simulink model "RealModelwithFlexibleLoad"  (R2019a)
settings: Solver=ode4  StartTime=0.0  StopTime=50.0  FixedStep=5e-5  MaxStep=1e-4  RelTol=1e-5
InitFcn:
  | Rs = 0.011
  | Ld = 0.018
  | Lq = 0.018
  | Fi = 0.055
  | p = 4
  | J = 0.002
  | b = 0.18
  | JL = 0.10
  | Bs = 0.00
  | Ks = 50
settings Model: Creator=LiLid  LastModifiedBy=LiLid

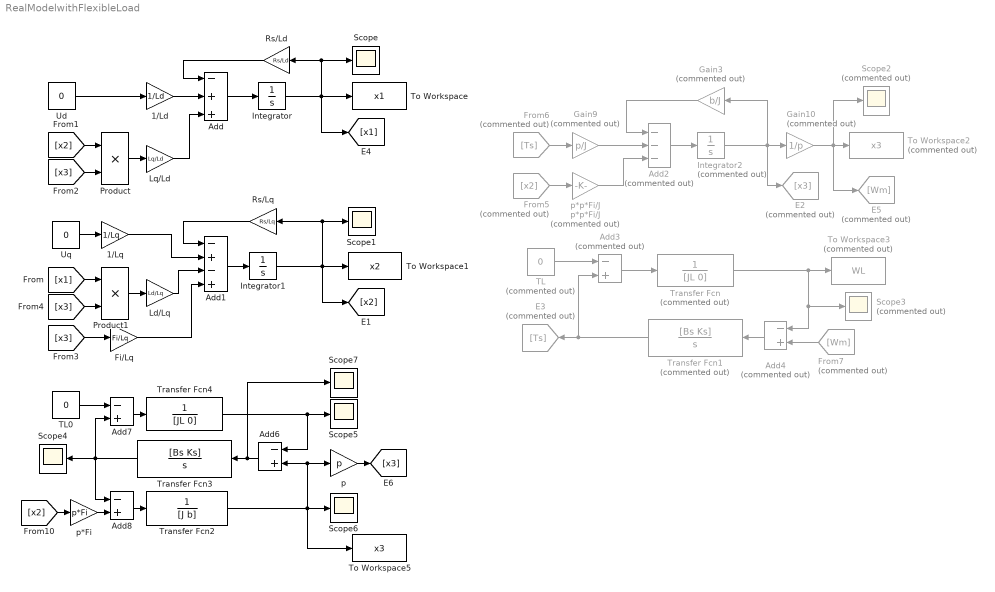
== system RealModelwithFlexibleLoad ==
  1/Ld : Gain  Gain=1/Ld
  1/Lq : Gain  Gain=1/Lq
  Add : Sum  Inputs=-++
  Add1 : Sum  Inputs=-+-+
  Add2 : Sum  Commented=on  Inputs=---
  Add3 : Sum  Commented=on  Inputs=-+
  Add4 : Sum  Commented=on  Inputs=-+
  Add6 : Sum  Inputs=-+
  Add7 : Sum  Inputs=-+
  Add8 : Sum  Inputs=-+
  E2 : Goto  Commented=on  GotoTag=x3
  E3 : Goto  Commented=on  GotoTag=Ts
  E5 : Goto  Commented=on  GotoTag=Wm
  Fi/Lq : Gain  Gain=Fi/Lq
  From5 : From  Commented=on  GotoTag=x2
  From6 : From  Commented=on  GotoTag=Ts
  From7 : From  Commented=on  GotoTag=Wm
  Gain10 : Gain  Commented=on  Gain=1/p
  Gain3 : Gain  Commented=on  Gain=b/J
  Gain9 : Gain  Commented=on  Gain=p/J
  Integrator : Integrator  InitialCondition=1
  Integrator1 : Integrator  InitialCondition=1
  Integrator2 : Integrator  Commented=on  InitialCondition=0.12
  Ld/Lq : Gain  Gain=Ld/Lq
  Lq/Ld : Gain  Gain=Lq/Ld
  Product : Product
  Product1 : Product
  Rs/Ld : Gain  Gain=Rs/Ld
  Rs/Lq : Gain  Gain=Rs/Lq
  Scope{,1,4..7} (6 alike) : Scope
  Scope2 : Scope  Commented=on
  Scope3 : Scope  Commented=on
  TL : Constant  Commented=on  Value=0
  TL0 : Constant  Value=0
  To Workspace : ToWorkspace  VariableName=x1  SampleTime=-1
      settings: Save2DSignal=2-D array (concatenate along first dimension)
  To Workspace1 : ToWorkspace  VariableName=x2  SampleTime=-1
      settings: Save2DSignal=2-D array (concatenate along first dimension)
  To Workspace2 : ToWorkspace  Commented=on  VariableName=x3  SampleTime=-1
      settings: Save2DSignal=2-D array (concatenate along first dimension)
  To Workspace3 : ToWorkspace  Commented=on  VariableName=WL  SampleTime=-1
      settings: Save2DSignal=2-D array (concatenate along first dimension)
  To Workspace5 : ToWorkspace  VariableName=x3  SampleTime=-1
      settings: Save2DSignal=2-D array (concatenate along first dimension)
  Transfer Fcn : TransferFcn  Commented=on  Denominator=[JL 0]
  Transfer Fcn1 : TransferFcn  Commented=on  Numerator=[Bs Ks]  Denominator=[1 0]
  Transfer Fcn2 : TransferFcn  Denominator=[J b]
  Transfer Fcn3 : TransferFcn  Numerator=[Bs Ks]  Denominator=[1 0]
  Transfer Fcn4 : TransferFcn  Denominator=[JL 0]
  Ud : Constant  Value=0
  Uq : Constant  Value=0
  p : Gain  Gain=p
  p*Fi : Gain  Gain=p*Fi
  p*p*Fi/J : Gain  Commented=on  Gain=p*p*Fi/J
  wires:
  Integrator/1 -> To Workspace/1, [x1], Scope/1, Rs/Ld/1
  Add/1 -> Integrator/1
  Rs/Ld/1 -> Add/1
  Product/1 -> Lq/Ld/1
  [x2] -> Product/1
  [x3] -> Product/2
  Integrator1/1 -> To Workspace1/1, Rs/Lq/1, Scope1/1, [x2]
  Rs/Lq/1 -> Add1/1
  Add1/1 -> Integrator1/1
  [x1] -> Product1/1
  [x3] -> Product1/2
  [x3] -> Fi/Lq/1
  Fi/Lq/1 -> Add1/4
  Integrator2/1 -> E2/1, Gain10/1, Gain3/1
  Add2/1 -> Integrator2/1
  Gain3/1 -> Add2/1
  From6/1 -> Gain9/1
  From5/1 -> p*p*Fi/J/1
  p*p*Fi/J/1 -> Add2/3
  Ud/1 -> 1/Ld/1
  Uq/1 -> 1/Lq/1
  Lq/Ld/1 -> Add/3
  1/Ld/1 -> Add/2
  1/Lq/1 -> Add1/2
  Product1/1 -> Ld/Lq/1
  Ld/Lq/1 -> Add1/3
  Gain9/1 -> Add2/2
  Gain10/1 -> Scope2/1, E5/1, To Workspace2/1
  Add3/1 -> Transfer Fcn/1
  TL/1 -> Add3/1
  Add4/1 -> Transfer Fcn1/1
  Transfer Fcn/1 -> To Workspace3/1, Scope3/1, Add4/1
  From7/1 -> Add4/2
  Transfer Fcn1/1 -> Add3/2, E3/1
  Add6/1 -> Scope7/1, Transfer Fcn3/1
  Transfer Fcn2/1 -> Scope6/1, Add6/2, p/1, To Workspace5/1
  Transfer Fcn4/1 -> Scope5/1, Add6/1
  Add7/1 -> Transfer Fcn4/1
  Transfer Fcn3/1 -> Add7/2, Scope4/1, Add8/1
  Add8/1 -> Transfer Fcn2/1
  p*Fi/1 -> Add8/2
  [x2] -> p*Fi/1
  TL0/1 -> Add7/1
  p/1 -> [x3]
